simulink subsystem "Node_wLocalObserver"  (R2024a)
settings: Solver=VariableStepAuto  StartTime=0.0  StopTime=10.0  RelTol=1e-3
values from neighbouring files (symbols this model uses):
  A = [0 1; 880.87 0]    [main.m]
  B = [0; -9.9453]    [main.m]
  C = [708.27 0]    [main.m]
  K0 = place(A, B, p_desired_tracking)    [main.m]
  Si_x0 = [0 0]'    [main.m]
undefined symbols (not defined in the file or in its folder): closed_loop_dynamics, closed_loop_local_observer
settings Model: Creator=Stefano  LastModifiedBy=Stefano

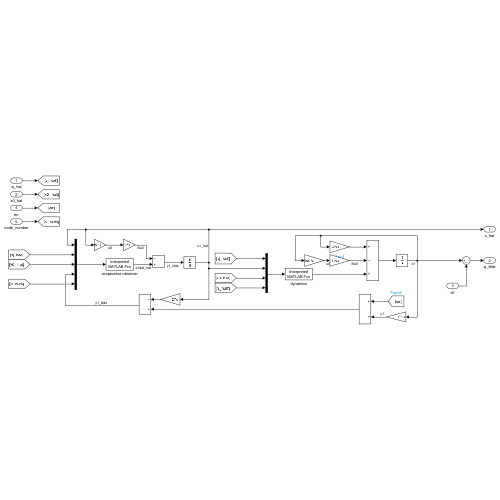
[thumbnail: Simulink's stored preview of the top-level diagram]
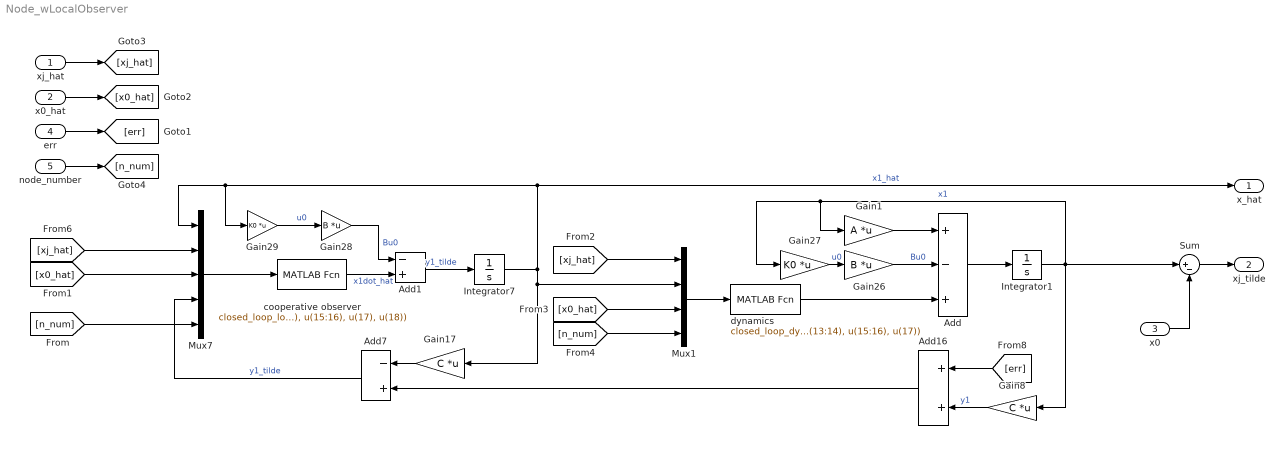
== system Node_wLocalObserver ==
  xj_hat : Inport
  x0_hat : Inport  Port=2
  x0 : Inport  Port=3
  err : Inport  Port=4
  node_number : Inport  Port=5
  Add : Sum  Inputs=+-+
  Add1 : Sum  Inputs=-+
  Add16 : Sum
  Add7 : Sum  Inputs=-+
  Gain1 : Gain  Gain=A  Multiplication=Matrix(K*u)
  Gain17 : Gain  Gain=C  Multiplication=Matrix(K*u)
  Gain26 : Gain  Gain=B  Multiplication=Matrix(K*u)
  Gain27 : Gain  Gain=K0  Multiplication=Matrix(K*u)
  Gain28 : Gain  Gain=B  Multiplication=Matrix(K*u)
  Gain29 : Gain  Gain=K0  Multiplication=Matrix(K*u)
  Gain8 : Gain  Gain=C  Multiplication=Matrix(K*u)
  Integrator1 : Integrator  InitialCondition=Si_x0
  Integrator7 : Integrator  InitialCondition=Si_x0
  Mux1 : Mux
  Mux7 : Mux  Inputs=5
  Sum : Sum  Inputs=|+-
  cooperative observer : MATLABFcn  MATLABFcn=closed_loop_local_observer(u(1:2), u(3:14), u(15:16), u(17), u(18))
  dynamics : MATLABFcn  MATLABFcn=closed_loop_dynamics(u(1:12), u(13:14), u(15:16), u(17))
  x_hat : Outport
  xj_tilde : Outport  Port=2
  wires:
  Gain8/1 -> Add16/2  "y1"
  [xj_hat] -> Mux1/1
  Mux7/1 -> cooperative observer/1
  Integrator7/1 -> Gain17/1, Mux1/2, x_hat/1, Gain29/1, Mux7/1  "x1_hat"
  dynamics/1 -> Add/3
  Gain17/1 -> Add7/1
  [x0_hat] -> Mux7/3
  Integrator1/1 -> Gain1/1, Gain27/1, Sum/1, Gain8/1  "x1"
  [x0_hat] -> Mux1/3
  Add7/1 -> Mux7/4  "y1_tilde"
  Gain1/1 -> Add/1
  [xj_hat] -> Mux7/2
  cooperative observer/1 -> Add1/2  "x1dot_hat"
  Add/1 -> Integrator1/1
  Mux1/1 -> dynamics/1
  x0_hat/1 -> [x0_hat]
  [n_num] -> Mux7/5
  xj_hat/1 -> [xj_hat]
  err/1 -> [err]
  [n_num] -> Mux1/4
  Sum/1 -> xj_tilde/1
  x0/1 -> Sum/2
  Gain29/1 -> Gain28/1  "u0"
  Add1/1 -> Integrator7/1  "y1_tilde"
  Gain28/1 -> Add1/1  "Bu0"
  Add16/1 -> Add7/2
  [err] -> Add16/1
  Gain26/1 -> Add/2  "Bu0"
  Gain27/1 -> Gain26/1  "u0"
  node_number/1 -> [n_num]
